simulink model "Msimlab3parte4"  (R2021a)
settings: Solver=VariableStepAuto  StartTime=0.0  StopTime=10  MaxStep=1e-4  RelTol=1e-3
values from neighbouring files (symbols this model uses):
  parede = 30    [p4_30.m]    (also in p4_60.m = 60; p4gif60.m = 60; p4gifs.m)
libraries: simulink x2
settings Model: Creator=danie  LastModifiedBy=ruipe
settings SolverCC: ZeroCrossAlgorithm=Adaptive  AlgebraicLoopSolver=TrustRegion
settings DebuggingCC: IgnoredZcDiagnostic=none  SFMachineParentedDataDiag=warning

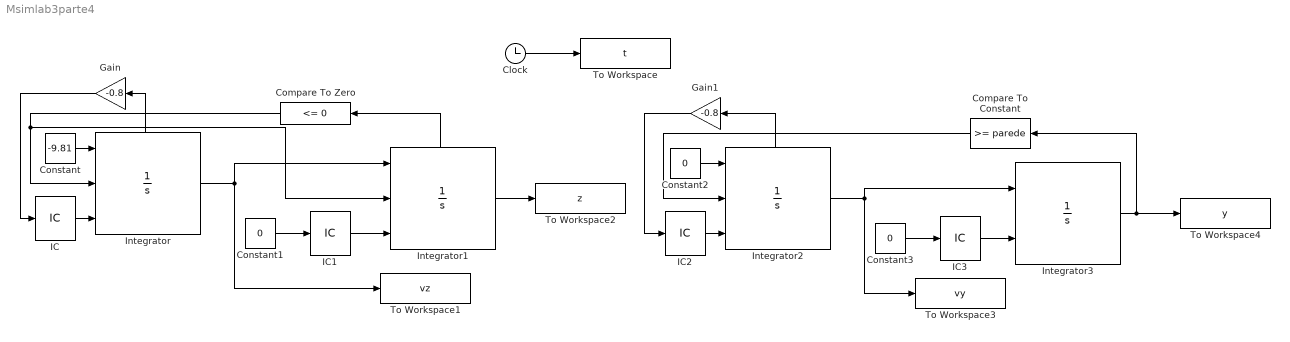
== system Msimlab3parte4 ==
  Clock : Clock
  Compare To Constant : simulink/Logic and Bit Operations/Compare To Constant  relop=>=  const=parede  OutDataTypeStr=boolean
  Compare To Zero : simulink/Logic and Bit Operations/Compare To Zero  relop=<=  OutDataTypeStr=boolean
  Constant : Constant  Description=Gravidade  Value=-9.81
      settings: AttributesFormatString=Gravidade
  Constant1 : Constant  Description=Pavimento  Value=0
      settings: AttributesFormatString=Pavimento
  Constant2 : Constant  Description=aceleração induzida em y  Value=0
  Constant3 : Constant  Description=Pavimento  Value=0
      settings: AttributesFormatString=Pavimento
  Gain : Gain  Description=Elasticidade da bola  Gain=-0.8
      settings: AttributesFormatString=Elasticidade da bola contra o chão
  Gain1 : Gain  Description=Elasticidade da bola  Gain=-0.8
      settings: AttributesFormatString=Elasticidade da bola contra a parede
  IC : InitialCondition  Description=Velocidade inicial  Value=0
      settings: AttributesFormatString=Velocidade inicial z
  IC1 : InitialCondition  Description=Posição inicial  Value=10
      settings: AttributesFormatString=Posição inicial z
  IC2 : InitialCondition  Description=Velocidade inicial  Value=10
      settings: AttributesFormatString=Velocidade inicial y
  IC3 : InitialCondition  Description=Posição inicial  Value=0
      settings: AttributesFormatString=Posição inicial y
  Integrator : Integrator  ExternalReset=level hold  InitialConditionSource=external  ShowStatePort=on
      settings: AttributesFormatString=Velocidade z
  Integrator1 : Integrator  ExternalReset=rising  InitialConditionSource=external  LimitOutput=on  ShowStatePort=on
      settings: AttributesFormatString=Posição z
  Integrator2 : Integrator  ExternalReset=level hold  InitialConditionSource=external  ShowStatePort=on
      settings: AttributesFormatString=Velocidade y
  Integrator3 : Integrator  InitialConditionSource=external  LimitOutput=on
      settings: AttributesFormatString=Posição y
  To Workspace : ToWorkspace  VariableName=t  SaveFormat=Timeseries  SampleTime=-1
      settings: Save2DSignal=2-D array (concatenate along first dimension)
  To Workspace1 : ToWorkspace  VariableName=vz  SaveFormat=Timeseries  SampleTime=-1
      settings: Save2DSignal=2-D array (concatenate along first dimension)
  To Workspace2 : ToWorkspace  VariableName=z  SaveFormat=Timeseries  SampleTime=-1
      settings: Save2DSignal=2-D array (concatenate along first dimension)
  To Workspace3 : ToWorkspace  VariableName=vy  SaveFormat=Timeseries  SampleTime=-1
      settings: Save2DSignal=2-D array (concatenate along first dimension)
  To Workspace4 : ToWorkspace  VariableName=y  SaveFormat=Timeseries  SampleTime=-1
      settings: Save2DSignal=2-D array (concatenate along first dimension)
  wires:
  Integrator1/1 -> To Workspace2/1
  Integrator1/State -> Compare To Zero/1
  Compare To Zero/1 -> Integrator/2, Integrator1/2
  Constant1/1 -> IC1/1
  IC1/1 -> Integrator1/3
  IC/1 -> Integrator/3
  Integrator/1 -> Integrator1/1, To Workspace1/1
  Clock/1 -> To Workspace/1
  Constant/1 -> Integrator/1
  Integrator/State -> Gain/1
  Gain/1 -> IC/1
  Integrator2/State -> Gain1/1
  Gain1/1 -> IC2/1
  Constant3/1 -> IC3/1
  Integrator3/1 -> To Workspace4/1, Compare To Constant/1
  Constant2/1 -> Integrator2/1
  IC2/1 -> Integrator2/3
  Compare To Constant/1 -> Integrator2/2
  IC3/1 -> Integrator3/2
  Integrator2/1 -> Integrator3/1, To Workspace3/1
